simulink model "gps"  (R2024a)
settings: configuration reference "standardSILConfiguraitonParams" (kept outside this file)
undefined symbols (not defined in the file): aircraftInitial, parameters
libraries: sensorgpslib x1
settings Model: Creator=GTAR  LastModifiedBy=jerem
settings ConfigSetRef: SourceName=standardSILConfiguraitonParams  SourceLocation=Base Workspace

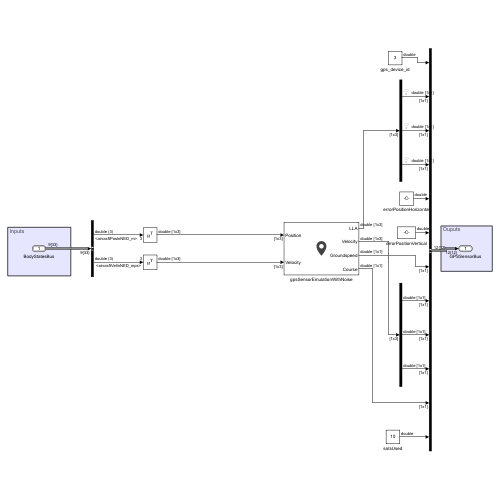
[thumbnail: Simulink's stored preview of the top-level diagram]
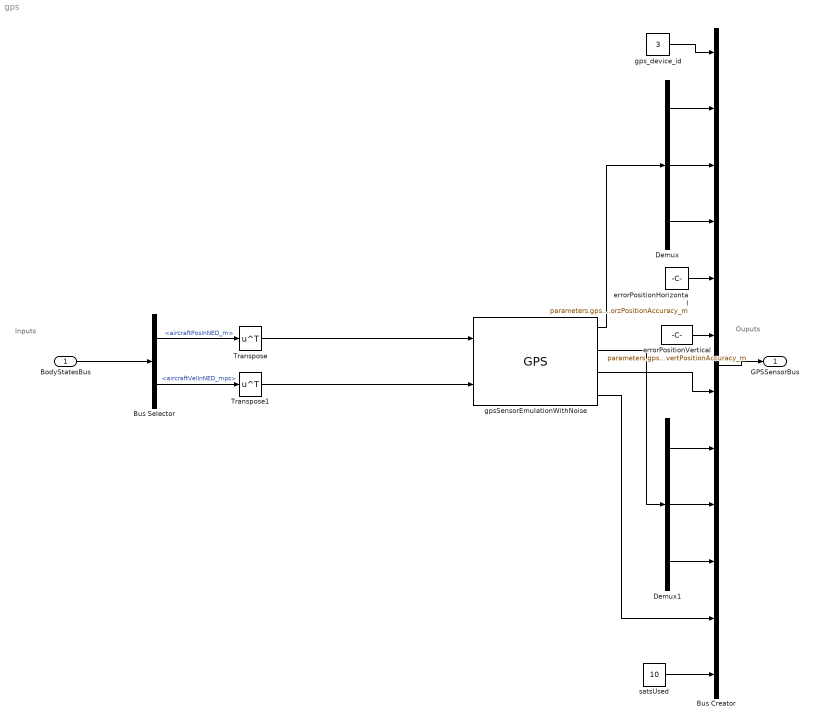
== system gps ==
  note: Ouputs
  note: Inputs
  BodyStatesBus : Inport  OutDataTypeStr=Bus: BodyStateBus
  Bus Creator : BusCreator  Inputs=12  OutDataTypeStr=Bus: GPSSensorBus
      settings: InheritFromInputs=off
  Bus Selector : BusSelector  OutputSignals=aircraftPosInNED_m,aircraftVelInNED_mps
  Demux : Demux  Outputs=3
  Demux1 : Demux  Outputs=3
  Transpose : Math  Operator=transpose
  Transpose1 : Math  Operator=transpose
  errorPositionHorizontal : Constant  Value=parameters.gps.horzPositionAccuracy_m  OutDataTypeStr=Inherit: Inherit via back propagation
  errorPositionVertical : Constant  Value=parameters.gps.vertPositionAccuracy_m  OutDataTypeStr=Inherit: Inherit via back propagation
  gpsSensorEmulationWithNoise : sensorgpslib/GPS  DispRefFrame=NED  PositionInputFormat=Local  ReferenceLocation=[ aircraftInitial.lat_deg, aircraftInitial.lon_deg, aircraftInitial.alt_m ]  HorizontalPositionAccuracy=0  VerticalPositionAccuracy=parameters.gps.vertPositionAccuracy_m  VelocityAccuracy=0  DecayFactor=0  SeedDouble=67  SimulateUsing=Interpreted execution
      settings: LibrarySourceBlock=uavsimlib/GPS
  gps_device_id : Constant  Value=3  OutDataTypeStr=double  LockScale=on
  satsUsed : Constant  Value=10  OutDataTypeStr=double
  GPSSensorBus : Outport  OutDataTypeStr=Bus: GPSSensorBus
  wires:
  errorPositionHorizontal/1 -> Bus Creator/5
  errorPositionVertical/1 -> Bus Creator/6
  satsUsed/1 -> Bus Creator/12
  Demux/1 -> Bus Creator/2
  Demux/2 -> Bus Creator/3
  Demux/3 -> Bus Creator/4
  Bus Creator/1 -> GPSSensorBus/1
  BodyStatesBus/1 -> Bus Selector/1
  Bus Selector/1 -> Transpose/1  "<aircraftPosInNED_m>"
  Bus Selector/2 -> Transpose1/1  "<aircraftVelInNED_mps>"
  gpsSensorEmulationWithNoise/3 -> Bus Creator/7
  gpsSensorEmulationWithNoise/1 -> Demux/1
  gpsSensorEmulationWithNoise/4 -> Bus Creator/11
  gpsSensorEmulationWithNoise/2 -> Demux1/1
  Demux1/1 -> Bus Creator/8
  Demux1/2 -> Bus Creator/9
  Demux1/3 -> Bus Creator/10
  gps_device_id/1 -> Bus Creator/1
  Transpose/1 -> gpsSensorEmulationWithNoise/1
  Transpose1/1 -> gpsSensorEmulationWithNoise/2
